simulink library "lib_TCML"  (R2015a)
settings: Solver=ode45  StartTime=0.0  StopTime=10.0  RelTol=1e-3
libraries: simulink x5
(part 7 of 7)

== matlab function lib_TCML/Dynamic Tip Clearance/Rotor Deformation/Deformation/Deformation Due To Thermal Expansion/Thermal Expansion 1D Elastic/MATLAB Function ==
  data: T_data input; L output; alpha_data input; Lo input; To input; Tf input; Erro input; BN input; Err output
function [L,Err] = ThermalExpansion(T_data,alpha_data,Lo,To,Tf,Erro,BN)
%#codegen

% initialize error/warning array
Err = Erro;
ErrNum = 1; %Error index

% number of data points for interpolation and numerical integration
n = 50;

%check input sizes
if length(T_data) < 2 && Erro(ErrNum) == 0
    Err(ErrNum) = 1;
    fprintf('warning in %s: The temperature data array (T_data) must be an array of at least 2 elements\n',char(BN));
end
ErrNum = ErrNum + 1;
if length(T_data) ~= length(alpha_data) && Erro(ErrNum) == 0
    Err(ErrNum) = 1;
    fprintf('warning in %s: The temperature data array (T_data) and corresponding thermal expansion coefficient data array (alpha_data) must be the same size\n',char(BN));
end
ErrNum = ErrNum + 1;
    
%check that To and Tf are in the range of T_data
if To < min(T_data)
    To = min(T_data);
    Err(ErrNum) = 1;
    if Erro(ErrNum) == 0
        fprintf('warning in %s: The previous/reference temperature (To) is less than the minimum value of the temperature data array T_data. Expand the data arrays to assure good results. The previous/reference temperature (To) has been set to the minimum value of T_data to avoid errors.\n',char(BN));
    end
end
ErrNum = ErrNum + 1;
if To > max(T_data)
    To = max(T_data);
    Err(ErrNum) = 1;
    if Erro(ErrNum) == 0
        fprintf('warning in %s: The previous/reference temperature (To) is greater than the maximum value of the temperature data array T_data. Expand the data arrays to assure good results. The previous/reference temperature (To) has been set to the maximum value of T_data to avoid errors.\n',char(BN));
    end
end
ErrNum = ErrNum + 1;
if Tf < min(T_data)
    Tf = min(T_data);
    Err(ErrNum) = 1;
    if Erro(ErrNum) == 0
        fprintf('warning in %s: The current temperature (Tf) is less than the minimum value of the temperature data array T_data. Expand the data arrays to assure good results. The current temperature (Tf) has been set to the maximum value of T_data to avoid errors.\n',char(BN));
    end
end
ErrNum = ErrNum + 1;
if Tf > max(T_data)
    Tf = max(T_data);
    Err(ErrNum) = 1;
    if Erro(ErrNum) == 0
        fprintf('warning in %s: The current temperature (Tf) is greater than the maximum value of the temperature data array T_data. Expand the data arrays to assure good results. The current temperature (Tf) has been set to the maximum value of T_data to avoid errors.\n',char(BN));
    end
end
ErrNum = ErrNum + 1;

%check that T_data is monotonically increasing
diffT = diff(T_data);
if min(diffT) <= 0 && Erro(ErrNum) == 0
    Err(ErrNum) = 1;
    fprintf('warning in %s: The temperature data array (T_data) must be monotonically increasing\n',char(BN));
end

T = linspace(To,Tf,n);
alpha = zeros(1,n);
for i = 1:n
    alpha(i) = interp1(T_data,alpha_data,T(i),'linear');
end

Int_alphadT = trapz(T,alpha);
dL = Lo*Int_alphadT;

L = Lo + dL;

== matlab function lib_TCML/Dynamic Tip Clearance/Rotor Deformation/Deformation1/Deformation Due To Thermal Expansion/Thermal Expansion 1D Elastic/MATLAB Function ==
  data: T_data input; L output; alpha_data input; Lo input; To input; Tf input; Erro input; BN input; Err output
function [L,Err] = ThermalExpansion(T_data,alpha_data,Lo,To,Tf,Erro,BN)
%#codegen

% initialize error/warning array
Err = Erro;
ErrNum = 1; %Error index

% number of data points for interpolation and numerical integration
n = 50;

%check input sizes
if length(T_data) < 2 && Erro(ErrNum) == 0
    Err(ErrNum) = 1;
    fprintf('warning in %s: The temperature data array (T_data) must be an array of at least 2 elements\n',char(BN));
end
ErrNum = ErrNum + 1;
if length(T_data) ~= length(alpha_data) && Erro(ErrNum) == 0
    Err(ErrNum) = 1;
    fprintf('warning in %s: The temperature data array (T_data) and corresponding thermal expansion coefficient data array (alpha_data) must be the same size\n',char(BN));
end
ErrNum = ErrNum + 1;
    
%check that To and Tf are in the range of T_data
if To < min(T_data)
    To = min(T_data);
    Err(ErrNum) = 1;
    if Erro(ErrNum) == 0
        fprintf('warning in %s: The previous/reference temperature (To) is less than the minimum value of the temperature data array T_data. Expand the data arrays to assure good results. The previous/reference temperature (To) has been set to the minimum value of T_data to avoid errors.\n',char(BN));
    end
end
ErrNum = ErrNum + 1;
if To > max(T_data)
    To = max(T_data);
    Err(ErrNum) = 1;
    if Erro(ErrNum) == 0
        fprintf('warning in %s: The previous/reference temperature (To) is greater than the maximum value of the temperature data array T_data. Expand the data arrays to assure good results. The previous/reference temperature (To) has been set to the maximum value of T_data to avoid errors.\n',char(BN));
    end
end
ErrNum = ErrNum + 1;
if Tf < min(T_data)
    Tf = min(T_data);
    Err(ErrNum) = 1;
    if Erro(ErrNum) == 0
        fprintf('warning in %s: The current temperature (Tf) is less than the minimum value of the temperature data array T_data. Expand the data arrays to assure good results. The current temperature (Tf) has been set to the maximum value of T_data to avoid errors.\n',char(BN));
    end
end
ErrNum = ErrNum + 1;
if Tf > max(T_data)
    Tf = max(T_data);
    Err(ErrNum) = 1;
    if Erro(ErrNum) == 0
        fprintf('warning in %s: The current temperature (Tf) is greater than the maximum value of the temperature data array T_data. Expand the data arrays to assure good results. The current temperature (Tf) has been set to the maximum value of T_data to avoid errors.\n',char(BN));
    end
end
ErrNum = ErrNum + 1;

%check that T_data is monotonically increasing
diffT = diff(T_data);
if min(diffT) <= 0 && Erro(ErrNum) == 0
    Err(ErrNum) = 1;
    fprintf('warning in %s: The temperature data array (T_data) must be monotonically increasing\n',char(BN));
end

T = linspace(To,Tf,n);
alpha = zeros(1,n);
for i = 1:n
    alpha(i) = interp1(T_data,alpha_data,T(i),'linear');
end

Int_alphadT = trapz(T,alpha);
dL = Lo*Int_alphadT;

L = Lo + dL;

== matlab function lib_TCML/Steady-State Tip Clearance/Case Deformation/While Iterator Subsystem2/MATLAB Function1 ==
  data: Tvec output; k input; Tavg output; W input; Tin input; hin input; Tout input; hout input
function [Tvec, Tavg] = SteadyStateTemp_Rotor(k,W,Tin,hin,Tout,hout)
%#codegen

B = [(hin+k/W) -k/W; -k/W (hout+k/W)]\[hin*Tin; hout*Tout];
Tavg = (B(1)+B(2))/2;

Tvec = [B(1) B(2)];

== matlab function lib_TCML/Steady-State Tip Clearance/Case Deformation/While Iterator Subsystem2/MATLAB Function2 ==
  data: Y_int output; X input; Y input; X_int input
function Y_int = interp1D(X,Y,X_int)
%#codegen

n = length(X);
if length(X) ~= length(Y)
    fprintf('warning: arrays for interpolating are not the same size\n');
end
if n < 2
    fprintf('warning: arrays for interpolating must at least 2 data points\n');
end
[rowX,colX] = size(X);
[rowY,colY] = size(Y);
if min([rowX,colX,rowY,colY]) > 1
    fprintf('warning: arrays for interpolating must be 1D arrays\n');
end
diffX = diff(X);
if min(diffX) <= 0
    fprintf('warning: the X array for interpolation must monotonically increasing\n');
end
real_X = isreal(X);
if min(real_X) == 0
    fprintf('warning: elements of X are not real\n');
end
real_Y = isreal(Y);
if min(real_Y) == 0
    fprintf('warning: elements of Y are not real\n');
end
real_Xint = isreal(X_int);
if min(real_Xint) == 0
    fprintf('warning: elements of X_int are not real\n');
end

N = length(X_int);
if min(X_int) < min(X)
    fprintf('warning: one or more element of X_int is lower than the range of X. The Y value corresponding to the minimum X will be output for Y_int in these cases.\n');
end
if max(X_int) > max(X)
    fprintf('warning: one or more element of X_int is higher than the range of X. The Y value corresponding to the maximmum X will be output for Y_int in these cases.\n');
end

Y_int = zeros(1,N);
for i = 1:N
    for j = 1:n-1
        if X_int(i) < X(1)
            Y_int(i) = Y(1);
            break
        elseif X_int(i) > X(end)
            Y_int(i) = Y(end);
            break
        elseif X_int(i) >= X(j) && X_int(i) <= X(j+1)
            Y_int(i) = (X_int(i) - X(j))/(X(j+1) - X(j))*(Y(j+1) - Y(j)) + Y(j);
            break
        end    
    end
end

== matlab function lib_TCML/Steady-State Tip Clearance/Case Deformation/Deformation/Thermal Expansion 1D Elastic/MATLAB Function ==
  data: T_data input; L output; alpha_data input; Lo input; To input; Tf input; Erro input; BN input; Err output
function [L,Err] = ThermalExpansion(T_data,alpha_data,Lo,To,Tf,Erro,BN)
%#codegen

% initialize error/warning array
Err = Erro;
ErrNum = 1; %Error index

% number of data points for interpolation and numerical integration
n = 50;

%check input sizes
if length(T_data) < 2 && Erro(ErrNum) == 0
    Err(ErrNum) = 1;
    fprintf('warning in %s: The temperature data array (T_data) must be an array of at least 2 elements\n',char(BN));
end
ErrNum = ErrNum + 1;
if length(T_data) ~= length(alpha_data) && Erro(ErrNum) == 0
    Err(ErrNum) = 1;
    fprintf('warning in %s: The temperature data array (T_data) and corresponding thermal expansion coefficient data array (alpha_data) must be the same size\n',char(BN));
end
ErrNum = ErrNum + 1;
    
%check that To and Tf are in the range of T_data
if To < min(T_data)
    To = min(T_data);
    Err(ErrNum) = 1;
    if Erro(ErrNum) == 0
        fprintf('warning in %s: The previous/reference temperature (To) is less than the minimum value of the temperature data array T_data. Expand the data arrays to assure good results. The previous/reference temperature (To) has been set to the minimum value of T_data to avoid errors.\n',char(BN));
    end
end
ErrNum = ErrNum + 1;
if To > max(T_data)
    To = max(T_data);
    Err(ErrNum) = 1;
    if Erro(ErrNum) == 0
        fprintf('warning in %s: The previous/reference temperature (To) is greater than the maximum value of the temperature data array T_data. Expand the data arrays to assure good results. The previous/reference temperature (To) has been set to the maximum value of T_data to avoid errors.\n',char(BN));
    end
end
ErrNum = ErrNum + 1;
if Tf < min(T_data)
    Tf = min(T_data);
    Err(ErrNum) = 1;
    if Erro(ErrNum) == 0
        fprintf('warning in %s: The current temperature (Tf) is less than the minimum value of the temperature data array T_data. Expand the data arrays to assure good results. The current temperature (Tf) has been set to the maximum value of T_data to avoid errors.\n',char(BN));
    end
end
ErrNum = ErrNum + 1;
if Tf > max(T_data)
    Tf = max(T_data);
    Err(ErrNum) = 1;
    if Erro(ErrNum) == 0
        fprintf('warning in %s: The current temperature (Tf) is greater than the maximum value of the temperature data array T_data. Expand the data arrays to assure good results. The current temperature (Tf) has been set to the maximum value of T_data to avoid errors.\n',char(BN));
    end
end
ErrNum = ErrNum + 1;

%check that T_data is monotonically increasing
diffT = diff(T_data);
if min(diffT) <= 0 && Erro(ErrNum) == 0
    Err(ErrNum) = 1;
    fprintf('warning in %s: The temperature data array (T_data) must be monotonically increasing\n',char(BN));
end

T = linspace(To,Tf,n);
alpha = zeros(1,n);
for i = 1:n
    alpha(i) = interp1(T_data,alpha_data,T(i),'linear');
end

Int_alphadT = trapz(T,alpha);
dL = Lo*Int_alphadT;

L = Lo + dL;

== matlab function lib_TCML/Dynamic Tip Clearance/Case Deformation/While Iterator Subsystem/MATLAB Function1 ==
  data: k input; Tavg output; W input; Tin input; hin input; Tout input; hout input
function Tavg = SteadyStateTemp_Rotor(k,W,Tin,hin,Tout,hout)
%#codegen

B = [(hin+k/W) -k/W; -k/W (hout+k/W)]\[hin*Tin; hout*Tout];
Tavg = (B(1)+B(2))/2;

== matlab function lib_TCML/Dynamic Tip Clearance/Rotor Deformation/While Iterator Subsystem/MATLAB Function1 ==
  data: k input; Tavg output; W input; Tin input; hin input; Tout input; hout input
function Tavg = SteadyStateTemp_Rotor(k,W,Tin,hin,Tout,hout)
%#codegen

B = [(hin+k/W) -k/W; -k/W (hout+k/W)]\[hin*Tin; hout*Tout];
Tavg = (B(1)+B(2))/2;

== matlab function lib_TCML/Steady-State Tip Clearance/Case Deformation/While Iterator Subsystem1/MATLAB Function1 ==
  data: Tvec output; k input; Tavg output; W input; Tin input; hin input; Tout input; hout input
function [Tvec, Tavg] = SteadyStateTemp_Rotor(k,W,Tin,hin,Tout,hout)
%#codegen

B = [(hin+k/W) -k/W; -k/W (hout+k/W)]\[hin*Tin; hout*Tout];
Tavg = (B(1)+B(2))/2;

Tvec = [B(1) B(2)];

== matlab function lib_TCML/Steady-State Tip Clearance/Case Deformation/While Iterator Subsystem1/MATLAB Function2 ==
  data: Y_int output; X input; Y input; X_int input
function Y_int = interp1D(X,Y,X_int)
%#codegen

n = length(X);
if length(X) ~= length(Y)
    fprintf('warning: arrays for interpolating are not the same size\n');
end
if n < 2
    fprintf('warning: arrays for interpolating must at least 2 data points\n');
end
[rowX,colX] = size(X);
[rowY,colY] = size(Y);
if min([rowX,colX,rowY,colY]) > 1
    fprintf('warning: arrays for interpolating must be 1D arrays\n');
end
diffX = diff(X);
if min(diffX) <= 0
    fprintf('warning: the X array for interpolation must monotonically increasing\n');
end
real_X = isreal(X);
if min(real_X) == 0
    fprintf('warning: elements of X are not real\n');
end
real_Y = isreal(Y);
if min(real_Y) == 0
    fprintf('warning: elements of Y are not real\n');
end
real_Xint = isreal(X_int);
if min(real_Xint) == 0
    fprintf('warning: elements of X_int are not real\n');
end

N = length(X_int);
if min(X_int) < min(X)
    fprintf('warning: one or more element of X_int is lower than the range of X. The Y value corresponding to the minimum X will be output for Y_int in these cases.\n');
end
if max(X_int) > max(X)
    fprintf('warning: one or more element of X_int is higher than the range of X. The Y value corresponding to the maximmum X will be output for Y_int in these cases.\n');
end

Y_int = zeros(1,N);
for i = 1:N
    for j = 1:n-1
        if X_int(i) < X(1)
            Y_int(i) = Y(1);
            break
        elseif X_int(i) > X(end)
            Y_int(i) = Y(end);
            break
        elseif X_int(i) >= X(j) && X_int(i) <= X(j+1)
            Y_int(i) = (X_int(i) - X(j))/(X(j+1) - X(j))*(Y(j+1) - Y(j)) + Y(j);
            break
        end    
    end
end

== matlab function lib_TCML/Steady-State Tip Clearance/Rotor Deformation/While Iterator Subsystem/MATLAB Function ==
  data: x output size=[1 2]; T output size=[1 2]; k input; Tavg output; W input; Tin input; hin input; Tout input; hout input
function [x,T,Tavg] = SteadyStateTemp_Rotor(k,W,Tin,hin,Tout,hout)
%#codegen

B = [(hin+k/W) -k/W; -k/W (hout+k/W)]\[hin*Tin; hout*Tout];

x = [0 W];
T = [B(1) B(2)];
Tavg = (B(1)+B(2))/2;

== matlab function lib_TCML/Steady-State Tip Clearance/Rotor Deformation/While Iterator Subsystem/MATLAB Function1 ==
  data: Y_int output; X input; Y input; X_int input
function Y_int = interp1D(X,Y,X_int)
%#codegen

n = length(X);
if length(X) ~= length(Y)
    fprintf('warning: arrays for interpolating are not the same size\n');
end
if n < 2
    fprintf('warning: arrays for interpolating must at least 2 data points\n');
end
[rowX,colX] = size(X);
[rowY,colY] = size(Y);
if min([rowX,colX,rowY,colY]) > 1
    fprintf('warning: arrays for interpolating must be 1D arrays\n');
end
diffX = diff(X);
if min(diffX) <= 0
    fprintf('warning: the X array for interpolation must monotonically increasing\n');
end
real_X = isreal(X);
if min(real_X) == 0
    fprintf('warning: elements of X are not real\n');
end
real_Y = isreal(Y);
if min(real_Y) == 0
    fprintf('warning: elements of Y are not real\n');
end
real_Xint = isreal(X_int);
if min(real_Xint) == 0
    fprintf('warning: elements of X_int are not real\n');
end

N = length(X_int);
if min(X_int) < min(X)
    fprintf('warning: one or more element of X_int is lower than the range of X. The Y value corresponding to the minimum X will be output for Y_int in these cases.\n');
end
if max(X_int) > max(X)
    fprintf('warning: one or more element of X_int is higher than the range of X. The Y value corresponding to the maximmum X will be output for Y_int in these cases.\n');
end

Y_int = zeros(1,N);
for i = 1:N
    for j = 1:n-1
        if X_int(i) < X(1)
            Y_int(i) = Y(1);
            break
        elseif X_int(i) > X(end)
            Y_int(i) = Y(end);
            break
        elseif X_int(i) >= X(j) && X_int(i) <= X(j+1)
            Y_int(i) = (X_int(i) - X(j))/(X(j+1) - X(j))*(Y(j+1) - Y(j)) + Y(j);
            break
        end    
    end
end

== matlab function lib_TCML/Steady-State Tip Clearance/Case Deformation/Deformation1/Thermal Expansion 1D Elastic/MATLAB Function ==
  data: T_data input; L output; alpha_data input; Lo input; To input; Tf input; Erro input; BN input; Err output
function [L,Err] = ThermalExpansion(T_data,alpha_data,Lo,To,Tf,Erro,BN)
%#codegen

% initialize error/warning array
Err = Erro;
ErrNum = 1; %Error index

% number of data points for interpolation and numerical integration
n = 50;

%check input sizes
if length(T_data) < 2 && Erro(ErrNum) == 0
    Err(ErrNum) = 1;
    fprintf('warning in %s: The temperature data array (T_data) must be an array of at least 2 elements\n',char(BN));
end
ErrNum = ErrNum + 1;
if length(T_data) ~= length(alpha_data) && Erro(ErrNum) == 0
    Err(ErrNum) = 1;
    fprintf('warning in %s: The temperature data array (T_data) and corresponding thermal expansion coefficient data array (alpha_data) must be the same size\n',char(BN));
end
ErrNum = ErrNum + 1;
    
%check that To and Tf are in the range of T_data
if To < min(T_data)
    To = min(T_data);
    Err(ErrNum) = 1;
    if Erro(ErrNum) == 0
        fprintf('warning in %s: The previous/reference temperature (To) is less than the minimum value of the temperature data array T_data. Expand the data arrays to assure good results. The previous/reference temperature (To) has been set to the minimum value of T_data to avoid errors.\n',char(BN));
    end
end
ErrNum = ErrNum + 1;
if To > max(T_data)
    To = max(T_data);
    Err(ErrNum) = 1;
    if Erro(ErrNum) == 0
        fprintf('warning in %s: The previous/reference temperature (To) is greater than the maximum value of the temperature data array T_data. Expand the data arrays to assure good results. The previous/reference temperature (To) has been set to the maximum value of T_data to avoid errors.\n',char(BN));
    end
end
ErrNum = ErrNum + 1;
if Tf < min(T_data)
    Tf = min(T_data);
    Err(ErrNum) = 1;
    if Erro(ErrNum) == 0
        fprintf('warning in %s: The current temperature (Tf) is less than the minimum value of the temperature data array T_data. Expand the data arrays to assure good results. The current temperature (Tf) has been set to the maximum value of T_data to avoid errors.\n',char(BN));
    end
end
ErrNum = ErrNum + 1;
if Tf > max(T_data)
    Tf = max(T_data);
    Err(ErrNum) = 1;
    if Erro(ErrNum) == 0
        fprintf('warning in %s: The current temperature (Tf) is greater than the maximum value of the temperature data array T_data. Expand the data arrays to assure good results. The current temperature (Tf) has been set to the maximum value of T_data to avoid errors.\n',char(BN));
    end
end
ErrNum = ErrNum + 1;

%check that T_data is monotonically increasing
diffT = diff(T_data);
if min(diffT) <= 0 && Erro(ErrNum) == 0
    Err(ErrNum) = 1;
    fprintf('warning in %s: The temperature data array (T_data) must be monotonically increasing\n',char(BN));
end

T = linspace(To,Tf,n);
alpha = zeros(1,n);
for i = 1:n
    alpha(i) = interp1(T_data,alpha_data,T(i),'linear');
end

Int_alphadT = trapz(T,alpha);
dL = Lo*Int_alphadT;

L = Lo + dL;

== matlab function lib_TCML/Steady-State Tip Clearance/Blade Deformation/Deformation/Deformation Due To Thermal Expansion/Thermal Expansion 1D Elastic/MATLAB Function ==
  data: T_data input; L output; alpha_data input; Lo input; To input; Tf input; Erro input; BN input; Err output
function [L,Err] = ThermalExpansion(T_data,alpha_data,Lo,To,Tf,Erro,BN)
%#codegen

% initialize error/warning array
Err = Erro;
ErrNum = 1; %Error index

% number of data points for interpolation and numerical integration
n = 50;

%check input sizes
if length(T_data) < 2 && Erro(ErrNum) == 0
    Err(ErrNum) = 1;
    fprintf('warning in %s: The temperature data array (T_data) must be an array of at least 2 elements\n',char(BN));
end
ErrNum = ErrNum + 1;
if length(T_data) ~= length(alpha_data) && Erro(ErrNum) == 0
    Err(ErrNum) = 1;
    fprintf('warning in %s: The temperature data array (T_data) and corresponding thermal expansion coefficient data array (alpha_data) must be the same size\n',char(BN));
end
ErrNum = ErrNum + 1;
    
%check that To and Tf are in the range of T_data
if To < min(T_data)
    To = min(T_data);
    Err(ErrNum) = 1;
    if Erro(ErrNum) == 0
        fprintf('warning in %s: The previous/reference temperature (To) is less than the minimum value of the temperature data array T_data. Expand the data arrays to assure good results. The previous/reference temperature (To) has been set to the minimum value of T_data to avoid errors.\n',char(BN));
    end
end
ErrNum = ErrNum + 1;
if To > max(T_data)
    To = max(T_data);
    Err(ErrNum) = 1;
    if Erro(ErrNum) == 0
        fprintf('warning in %s: The previous/reference temperature (To) is greater than the maximum value of the temperature data array T_data. Expand the data arrays to assure good results. The previous/reference temperature (To) has been set to the maximum value of T_data to avoid errors.\n',char(BN));
    end
end
ErrNum = ErrNum + 1;
if Tf < min(T_data)
    Tf = min(T_data);
    Err(ErrNum) = 1;
    if Erro(ErrNum) == 0
        fprintf('warning in %s: The current temperature (Tf) is less than the minimum value of the temperature data array T_data. Expand the data arrays to assure good results. The current temperature (Tf) has been set to the maximum value of T_data to avoid errors.\n',char(BN));
    end
end
ErrNum = ErrNum + 1;
if Tf > max(T_data)
    Tf = max(T_data);
    Err(ErrNum) = 1;
    if Erro(ErrNum) == 0
        fprintf('warning in %s: The current temperature (Tf) is greater than the maximum value of the temperature data array T_data. Expand the data arrays to assure good results. The current temperature (Tf) has been set to the maximum value of T_data to avoid errors.\n',char(BN));
    end
end
ErrNum = ErrNum + 1;

%check that T_data is monotonically increasing
diffT = diff(T_data);
if min(diffT) <= 0 && Erro(ErrNum) == 0
    Err(ErrNum) = 1;
    fprintf('warning in %s: The temperature data array (T_data) must be monotonically increasing\n',char(BN));
end

T = linspace(To,Tf,n);
alpha = zeros(1,n);
for i = 1:n
    alpha(i) = interp1(T_data,alpha_data,T(i),'linear');
end

Int_alphadT = trapz(T,alpha);
dL = Lo*Int_alphadT;

L = Lo + dL;

== matlab function lib_TCML/Steady-State Tip Clearance/Rotor Deformation/Deformation/Deformation Due To Thermal Expansion/Thermal Expansion 1D Elastic/MATLAB Function ==
  data: T_data input; L output; alpha_data input; Lo input; To input; Tf input; Erro input; BN input; Err output
function [L,Err] = ThermalExpansion(T_data,alpha_data,Lo,To,Tf,Erro,BN)
%#codegen

% initialize error/warning array
Err = Erro;
ErrNum = 1; %Error index

% number of data points for interpolation and numerical integration
n = 50;

%check input sizes
if length(T_data) < 2 && Erro(ErrNum) == 0
    Err(ErrNum) = 1;
    fprintf('warning in %s: The temperature data array (T_data) must be an array of at least 2 elements\n',char(BN));
end
ErrNum = ErrNum + 1;
if length(T_data) ~= length(alpha_data) && Erro(ErrNum) == 0
    Err(ErrNum) = 1;
    fprintf('warning in %s: The temperature data array (T_data) and corresponding thermal expansion coefficient data array (alpha_data) must be the same size\n',char(BN));
end
ErrNum = ErrNum + 1;
    
%check that To and Tf are in the range of T_data
if To < min(T_data)
    To = min(T_data);
    Err(ErrNum) = 1;
    if Erro(ErrNum) == 0
        fprintf('warning in %s: The previous/reference temperature (To) is less than the minimum value of the temperature data array T_data. Expand the data arrays to assure good results. The previous/reference temperature (To) has been set to the minimum value of T_data to avoid errors.\n',char(BN));
    end
end
ErrNum = ErrNum + 1;
if To > max(T_data)
    To = max(T_data);
    Err(ErrNum) = 1;
    if Erro(ErrNum) == 0
        fprintf('warning in %s: The previous/reference temperature (To) is greater than the maximum value of the temperature data array T_data. Expand the data arrays to assure good results. The previous/reference temperature (To) has been set to the maximum value of T_data to avoid errors.\n',char(BN));
    end
end
ErrNum = ErrNum + 1;
if Tf < min(T_data)
    Tf = min(T_data);
    Err(ErrNum) = 1;
    if Erro(ErrNum) == 0
        fprintf('warning in %s: The current temperature (Tf) is less than the minimum value of the temperature data array T_data. Expand the data arrays to assure good results. The current temperature (Tf) has been set to the maximum value of T_data to avoid errors.\n',char(BN));
    end
end
ErrNum = ErrNum + 1;
if Tf > max(T_data)
    Tf = max(T_data);
    Err(ErrNum) = 1;
    if Erro(ErrNum) == 0
        fprintf('warning in %s: The current temperature (Tf) is greater than the maximum value of the temperature data array T_data. Expand the data arrays to assure good results. The current temperature (Tf) has been set to the maximum value of T_data to avoid errors.\n',char(BN));
    end
end
ErrNum = ErrNum + 1;

%check that T_data is monotonically increasing
diffT = diff(T_data);
if min(diffT) <= 0 && Erro(ErrNum) == 0
    Err(ErrNum) = 1;
    fprintf('warning in %s: The temperature data array (T_data) must be monotonically increasing\n',char(BN));
end

T = linspace(To,Tf,n);
alpha = zeros(1,n);
for i = 1:n
    alpha(i) = interp1(T_data,alpha_data,T(i),'linear');
end

Int_alphadT = trapz(T,alpha);
dL = Lo*Int_alphadT;

L = Lo + dL;
